simulink model "Klademodel"  (R2024a)
settings: Solver=VariableStepAuto  StartTime=0.0  StopTime=100  RelTol=1e-3
undefined symbols (not defined in the file or in its folder): Deq, Jeq, Kt, n, Ra
settings Model: Creator=jesperbertelsen  LastModifiedBy=jesperbertelsen

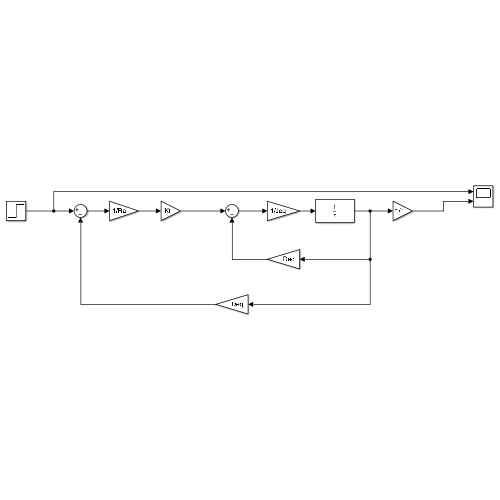
[thumbnail: Simulink's stored preview of the top-level diagram]
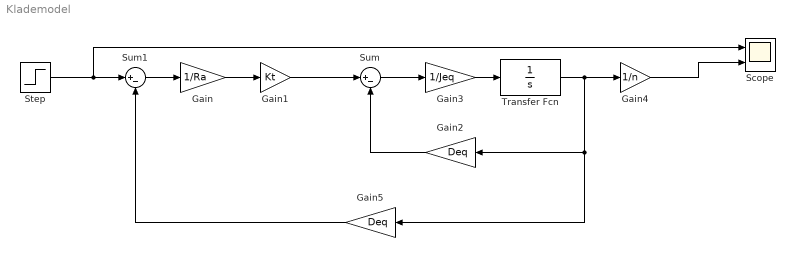
== system Klademodel ==
  Gain : Gain  Gain=1/Ra
  Gain1 : Gain  Gain=Kt
  Gain2 : Gain  Gain=Deq
  Gain3 : Gain  Gain=1/Jeq
  Gain4 : Gain  Gain=1/n
  Gain5 : Gain  Gain=Deq
  Scope : Scope  NumInputPorts=2
  Step : Step  After=5  SampleTime=0
  Sum : Sum  Inputs=|+-
  Sum1 : Sum  Inputs=|+-
  Transfer Fcn : TransferFcn  Denominator=[1 0]
  wires:
  Gain/1 -> Gain1/1
  Sum1/1 -> Gain/1
  Gain1/1 -> Sum/1
  Gain2/1 -> Sum/2
  Sum/1 -> Gain3/1
  Gain3/1 -> Transfer Fcn/1
  Transfer Fcn/1 -> Gain4/1, Gain5/1, Gain2/1
  Step/1 -> Scope/1, Sum1/1
  Gain4/1 -> Scope/2
  Gain5/1 -> Sum1/2
